simulink model "floating_point_simulink"  (Simulink 7.8)
settings: Solver=VariableStepDiscrete  StartTime=0.0  StopTime=1  RelTol=1e-3
settings Model: Creator=chuh  LastModifiedBy=chuh

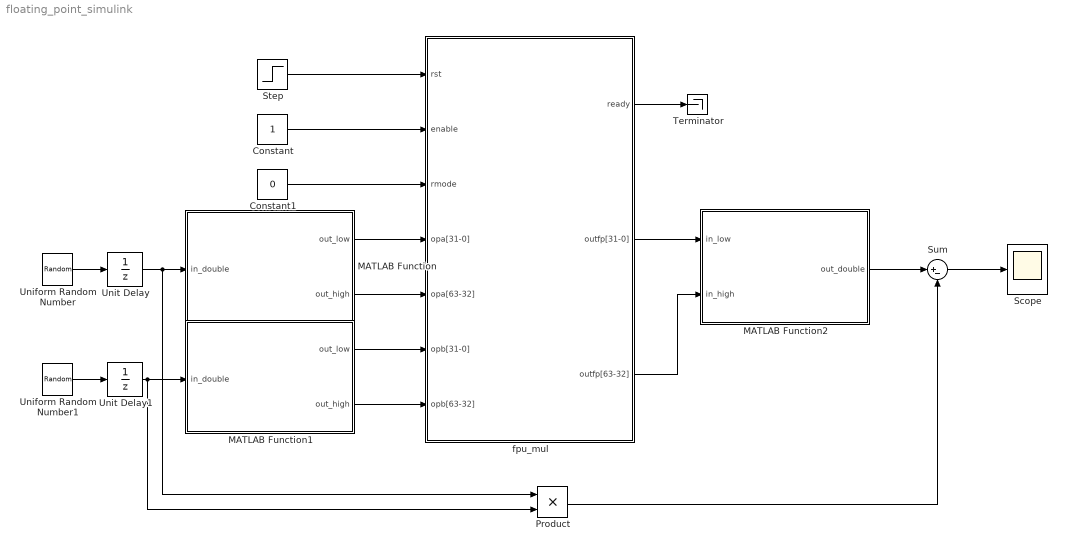
== system floating_point_simulink ==
  Constant : Constant
  Constant1 : Constant  Value=0
  MATLAB Function : MATLAB Function  TreatAsAtomicUnit=on
  MATLAB Function1 : MATLAB Function  TreatAsAtomicUnit=on
  MATLAB Function2 : MATLAB Function  TreatAsAtomicUnit=on
  Product : Product  RndMeth=Zero
  Scope : Scope
      settings: YMin=-7  YMax=10  SaveName=sim_error  SampleInput=on  SampleTime=0.001
  Step : Step  Time=0.002  Before=1  After=0  SampleTime=0
  Sum : Sum  Inputs=|+-
  Terminator : Terminator
  Uniform Random Number : UniformRandomNumber  Minimum=-2^307  Maximum=2^307  SampleTime=0.001
  Uniform Random Number1 : UniformRandomNumber  Minimum=-2^307  Maximum=2^307  SampleTime=0.001
  Unit Delay : UnitDelay  SampleTime=0.002
  Unit Delay1 : UnitDelay  SampleTime=0.002
  fpu_mul : Subsystem  mask(fpu_mul){params_samples=0.001, params_freq=50}
      mask prompts: params_samples "Sample time:"; params_freq "FPGA frequency (MHz):"
      mask help:
      | input rst
      | input enable
      | input rmode[1:0]
      | input opa[63:0]
      | input opb[63:0]
      | output ready
      | output outfp[63:0]
      mask Help:
      | input rst
      | input enable
      | input rmode[1:0]
      | input opa[63:0]
      | input opb[63:0]
      | output ready
      | output outfp[63:0]
  wires:
  Step/1 -> fpu_mul/1(rst)
  Constant/1 -> fpu_mul/2(enable)
  Constant1/1 -> fpu_mul/3(rmode)
  MATLAB Function/1(out_low) -> fpu_mul/4(opa[31-0])
  MATLAB Function/2(out_high) -> fpu_mul/5(opa[63-32])
  MATLAB Function1/1(out_low) -> fpu_mul/6(opb[31-0])
  MATLAB Function1/2(out_high) -> fpu_mul/7(opb[63-32])
  fpu_mul/1(ready) -> Terminator/1
  fpu_mul/2(outfp[31-0]) -> MATLAB Function2/1(in_low)
  fpu_mul/3(outfp[63-32]) -> MATLAB Function2/2(in_high)
  MATLAB Function2/1(out_double) -> Sum/1
  Uniform Random Number/1 -> Unit Delay/1
  Uniform Random Number1/1 -> Unit Delay1/1
  Unit Delay/1 -> MATLAB Function/1(in_double), Product/1
  Unit Delay1/1 -> MATLAB Function1/1(in_double), Product/2
  Sum/1 -> Scope/1
  Product/1 -> Sum/2

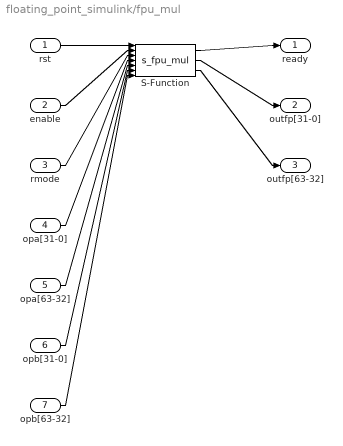
== system floating_point_simulink/fpu_mul ==
  rst : Inport  OutDataTypeStr=double  SampleTime=0.001
  enable : Inport  Port=2  OutDataTypeStr=double  SampleTime=0.001
  rmode : Inport  Port=3  OutDataTypeStr=double  SampleTime=0.001
  opa[31-0] : Inport  Port=4  OutDataTypeStr=double  SampleTime=0.001
  opa[63-32] : Inport  Port=5  OutDataTypeStr=double  SampleTime=0.001
  opb[31-0] : Inport  Port=6  OutDataTypeStr=double  SampleTime=0.001
  opb[63-32] : Inport  Port=7  OutDataTypeStr=double  SampleTime=0.001
  S-Function : S-Function  FunctionName=s_fpu_mul  Parameters=params_samples, params_freq  EnableBusSupport=off
  ready : Outport  OutDataTypeStr=uint32  SampleTime=0.001
  outfp[31-0] : Outport  Port=2  OutDataTypeStr=uint32  SampleTime=0.001
  outfp[63-32] : Outport  Port=3  OutDataTypeStr=uint32  SampleTime=0.001
  wires:
  rst/1 -> S-Function/1
  enable/1 -> S-Function/2
  rmode/1 -> S-Function/3
  opa[31-0]/1 -> S-Function/4
  opa[63-32]/1 -> S-Function/5
  opb[31-0]/1 -> S-Function/6
  opb[63-32]/1 -> S-Function/7
  S-Function/1 -> ready/1
  S-Function/2 -> outfp[31-0]/1
  S-Function/3 -> outfp[63-32]/1

== matlab function MATLAB Function1 ==
  data: in_double input double; out_low output double; out_high output double
function [out_low, out_high] = fcn(in_double)

x=typecast(in_double,'uint32');

out_low=double(x(1));
out_high=double(x(2));

== matlab function MATLAB Function ==
  data: in_double input double; out_low output double; out_high output double
function [out_low, out_high] = fcn(in_double)

x=typecast(in_double,'uint32');

out_low=double(x(1));
out_high=double(x(2));

== matlab function MATLAB Function2 ==
  data: in_low input uint32; out_double output double; in_high input uint32
function out_double  = fcn(in_low, in_high)

out_double=typecast([in_low; in_high],'double');
